simulink model "F550_verify_trim"  (R2024a)
settings: Solver=VariableStepAuto  StartTime=0.0  StopTime=100  FixedStep=0.001  RelTol=1e-3
values from neighbouring files (symbols this model uses):
  r2d = 180/pi    (= 57.2957795131)    [F550_data.m]
  u0 = opreport.inputs.u    [trim_F550_model.m]
settings Model: Creator=ADMIN  LastModifiedBy=CNU_UASG
settings DataIOCC: ExternalInput=getinputstruct(op_trim1)  InitialState=getstatestruct(op_trim1)
settings DebuggingCC: UnconnectedInputMsg=warning  UnconnectedOutputMsg=warning  UnconnectedLineMsg=warning
settings ModelReferenceCC: EnableRefExpFcnMdlSchedulingChecks=on
settings RTWCC: GPUComputeCapability=3.5  DLArmComputeVersion=19.05

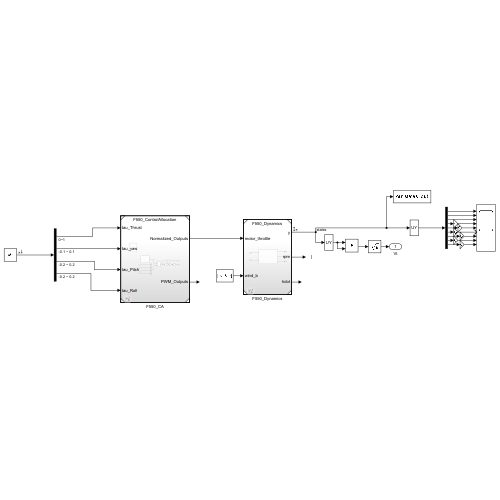
[thumbnail: Simulink's stored preview of the top-level diagram]
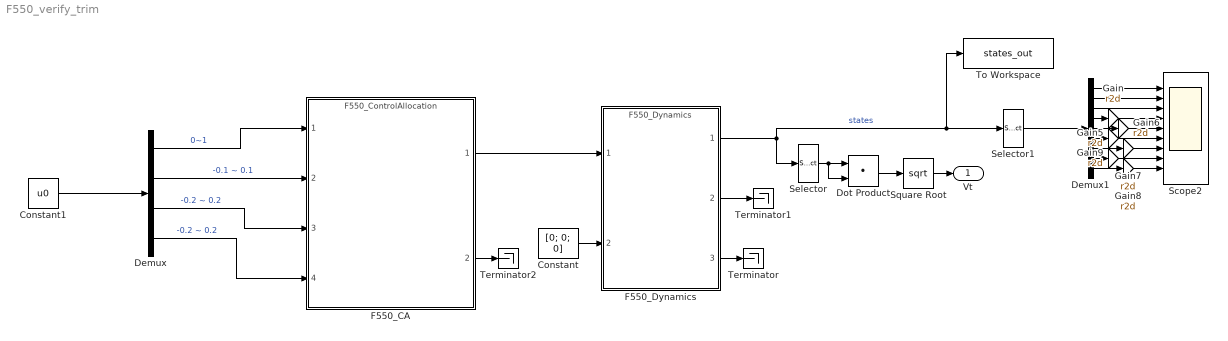
== system F550_verify_trim ==
  Constant : Constant  Value=[0; 0; 0]
  Constant1 : Constant  Value=u0
  Demux : Demux
  Demux1 : Demux  Outputs=9
  Dot Product : DotProduct  OutDataTypeStr=Inherit: Inherit via internal rule
  F550_CA : ModelReference  ModelNameDialog=F550_ControlAllocation.slx  SimulationMode=Normal  ModelReferenceVersion=1.8
  F550_Dynamics : ModelReference  ModelNameDialog=F550_Dynamics.slx  SimulationMode=Normal  ModelReferenceVersion=1.10
  Gain{,5..9} (6 alike) : Gain  Gain=r2d
  Scope2 : Scope  NumInputPorts=9
  Selector : Selector  InputPortWidth=12  IndexOptions=Index vector (dialog)  Indices=[1 2 3]  OutputSizes=1
  Selector1 : Selector  InputPortWidth=12  IndexOptions=Index vector (dialog)  Indices=1:9  OutputSizes=1
  Square Root : Sqrt
  Terminator : Terminator
  Terminator1 : Terminator
  Terminator2 : Terminator
  To Workspace : ToWorkspace  VariableName=states_out  SampleTime=-1
  Vt : Outport
  wires:
  Demux/4 -> F550_CA/4  "-0.2 ~ 0.2"
  Demux/3 -> F550_CA/3  "-0.2 ~ 0.2"
  Demux/2 -> F550_CA/2  "-0.1 ~ 0.1"
  Demux/1 -> F550_CA/1  "0~1"
  Selector/1 -> Dot Product/1, Dot Product/2
  Square Root/1 -> Vt/1
  Dot Product/1 -> Square Root/1
  F550_Dynamics/1 -> Selector/1, Selector1/1, To Workspace/1  "states"
  F550_Dynamics/3 -> Terminator/1
  Constant/1 -> F550_Dynamics/2
  F550_CA/1 -> F550_Dynamics/1
  F550_CA/2 -> Terminator2/1
  Constant1/1 -> Demux/1
  F550_Dynamics/2 -> Terminator1/1
  Gain5/1 -> Scope2/6
  Demux1/9 -> Gain8/1
  Demux1/7 -> Gain7/1
  Demux1/3 -> Scope2/3
  Demux1/1 -> Scope2/1
  Demux1/2 -> Scope2/2
  Demux1/4 -> Gain/1
  Gain8/1 -> Scope2/9
  Gain7/1 -> Scope2/7
  Demux1/8 -> Gain9/1
  Selector1/1 -> Demux1/1
  Demux1/5 -> Gain6/1
  Gain/1 -> Scope2/4
  Gain6/1 -> Scope2/5
  Gain9/1 -> Scope2/8
  Demux1/6 -> Gain5/1
